simulink model "ee_import_fem_maxwell"  (R2021b)
settings: Solver=FixedStepAuto  StartTime=0.0  StopTime=tsim  FixedStep=Ts  RelTol=1e-3  AbsTol=1e-3
StopFcn:
  | ee_addSimlogTimeStamp(bdroot)
values from neighbouring files (symbols this model uses):
  angleVec = [0 1 2 3 4 5 6 7 8 9 10 11 ... (31 elements, 1x31)]    [matlab.mat]
  data =     [pmsm_phi2i_21p.mat]
  fdVec = Phid_Vec(index_d)    [di_pmsm_model_generator_invLUT_V2.m]    (also in matlab.mat = [-0.2 -0.175 -0.15 -0.125 -0.1 0 0.1 0.15 0.2 0.25 0.3])
  fqVec = Phiq_Vec(index_q)    [di_pmsm_model_generator_invLUT_V2.m]    (also in matlab.mat = [-0.3 -0.24 -0.18 -0.12 -0.09 0 0.09 0.12 0.18 0.24 0.3])
  Id_LUT = Id_perm(:,index_d,index_q)    [di_pmsm_model_generator_invLUT_V2.m]    (also in matlab.mat = [-299.999952118 -299.999957203 -299.999957203 -299.999957203)
  Id_orig = fliplr(data.i_d)    [di_pmsm_model_generator_invLUT_V2.m]
  Iq_LUT = Iq_perm(:,index_d,index_q)    [di_pmsm_model_generator_invLUT_V2.m]    (also in matlab.mat = [-180.584816304 -190.608960928 -197.843546268 -189.111216324)
  Iq_orig = fliplr(-data.i_q)    [di_pmsm_model_generator_invLUT_V2.m]
  J = 0.02    [di_pmsm_model_MPC_ideal_k2.m]    (also in di_pmsm_model_MPC_k1.m; di_pmsm_model_MPC_k2.m; di_pmsm_model_generator_invLUT_V2.m)
  Ld = 0.0013    [di_pmsm_model_MPC_ideal_k2.m]    (also in di_pmsm_model_MPC_k1.m; di_pmsm_model_MPC_k2.m; di_pmsm_model_generator_invLUT_V2.m)
  Lq = 0.0039    [di_pmsm_model_MPC_ideal_k2.m]    (also in di_pmsm_model_MPC_k1.m; di_pmsm_model_MPC_k2.m; di_pmsm_model_generator_invLUT_V2.m)
  omegae = omegae_ref    [di_pmsm_model_MPC_ideal_k2.m]    (also in di_pmsm_model_MPC_k1.m; di_pmsm_model_MPC_k2.m; di_pmsm_model_generator_invLUT_V2.m = N*RPM*2*pi/60)
  PM = 0.1571    [di_pmsm_model_MPC_ideal_k2.m]    (also in di_pmsm_model_MPC_k1.m; di_pmsm_model_MPC_k2.m; di_pmsm_model_generator_invLUT_V2.m)
  R_s = 0.07    [di_pmsm_model_MPC_ideal_k2.m]    (also in di_pmsm_model_MPC_k1.m; di_pmsm_model_MPC_k2.m; di_pmsm_model_generator_invLUT_V2.m)
  RPM = 1000    [di_pmsm_model_generator_invLUT_V2.m]    (also in sim_3f_fcsmpc_k1.m = 3000)
  torque = fliplr(torque)    [param_fcsmpc.m]    (also in sim_3f_fcsmpc_k1.m = tray_sim_par_real(1:param_sim_Nh))
  Torque_orig = fliplr(torque)    [di_pmsm_model_generator_invLUT_V2.m]
  Torque_perm = permute(Torque_orig,[3,1,2])    [di_pmsm_model_generator_invLUT_V2.m]    (also in matlab.mat = [-417.44568224 -399.66222402 -374.4267079 -354.35960705 -348)
undefined symbols (not defined in the file or in its folder): idVec, iqVec, N
CloseFcn:
  | try,close(h1_ee_import_fem_maxwell),end
  | clear h1_ee_import_fem_maxwell
  | clear simlog_ee_import_fem_maxwell
  | clear N RPM Rload
  | clear angleVec idVec iqVec
  | clear flux0 fluxD fluxQ
  | clear torque
Description:
  | Import IPMSM Flux Linkage Data from ANSYS Maxwell
settings Model: Creator=The MathWorks, Inc.  LastModifiedBy=crist
settings SolverCC: AutoScaleAbsTol=off  AlgebraicLoopSolver=TrustRegion
settings DataIOCC: SaveOutput=off  SignalLogging=off  DSMLogging=off  SaveTime=off  ReturnWorkspaceOutputs=off
settings DebuggingCC: SFMachineParentedDataDiag=warning  ArithmeticOperatorsInVariantConditions=warning
settings SFSimCC: SimUseLocalCustomCode=off  CustomCodeUndefinedFunction=UseInterfaceOnly
settings RTWCC: RTWUseLocalCustomCode=off
settings SimscapeCC: SimscapeLogType=all  SimscapeLogName=simlog_ee_import_fem_maxwell  SimscapeLogLimitData=off  SimscapeLogDataHistory=50000

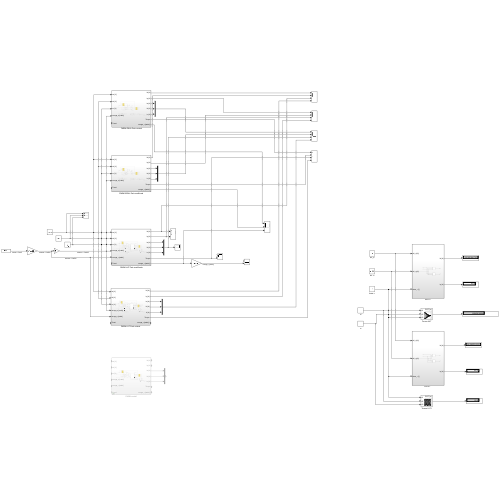
[thumbnail: Simulink's stored preview of the top-level diagram]
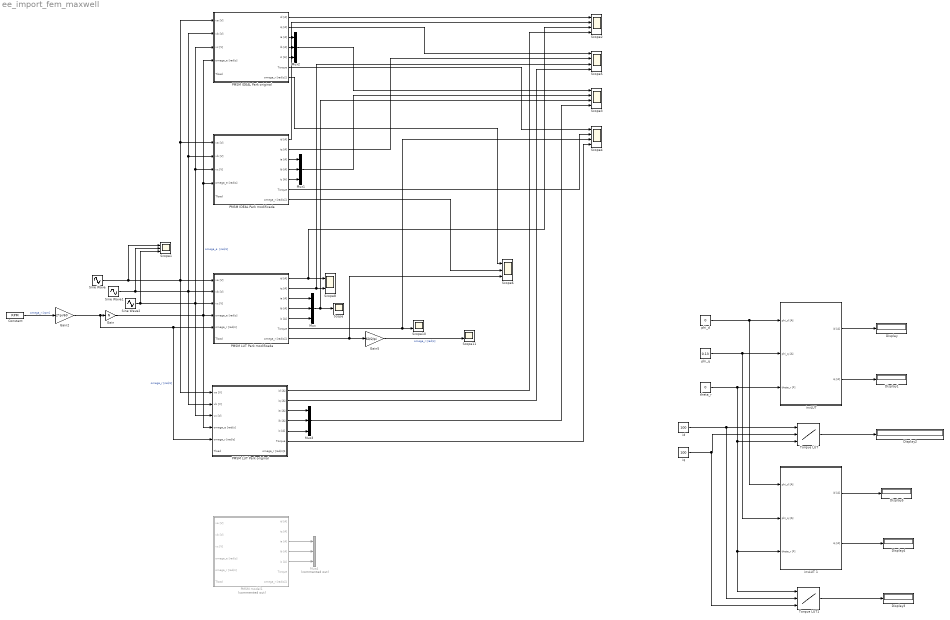
== system ee_import_fem_maxwell ==
  Constant : Constant  Value=RPM
  Display{,1..5} (6 alike) : Display
  Gain : Gain  Gain=N
  Gain2 : Gain  Gain=2*pi/60
  Gain5 : Gain  Gain=60/2/pi
  Mux{,1..3} (4 alike) : Mux  Inputs=3
  Mux4 : Mux  Commented=on  Inputs=3
  PMSM IDEAL Park modificada : Subsystem
  PMSM IDEAL Park original : Subsystem
  PMSM LUT Park modificada : Subsystem
  PMSM LUT Park original : Subsystem
  PMSM model1 : Subsystem  Commented=on
  Scope : Scope
  Scope1 : Scope  NumInputPorts=3
  Scope10 : Scope  NumInputPorts=2
  Scope11 : Scope  NumInputPorts=2
  Scope{2..5} (4 alike) : Scope  NumInputPorts=4
  Scope6 : Scope  NumInputPorts=3
  Scope8 : Scope  NumInputPorts=2
  Sine Wave : Sin  Amplitude=10  Frequency=omegae  Phase=pi/2  SampleTime=0
  Sine Wave1 : Sin  Amplitude=10  Frequency=omegae  Phase=-2*pi/3+pi/2  SampleTime=0
  Sine Wave2 : Sin  Amplitude=10  Frequency=omegae  Phase=-4*pi/3+pi/2  SampleTime=0
  Torque LUT : Lookup_n-D  NumberOfTableDimensions=3  LookupTableObject=iD  BreakpointsForDimension1=idVec  BreakpointsForDimension2=iqVec  BreakpointsForDimension3=angleVec  Table=Torque_orig  InternalRulePriority=Speed  RndMeth=Simplest  InputSameDT=on
      settings: InputPortMap=u0,u1,u2
  Torque LUT1 : Lookup_n-D  NumberOfTableDimensions=3  LookupTableObject=iD  BreakpointsForDimension1=angleVec  BreakpointsForDimension2=idVec  BreakpointsForDimension3=iqVec  Table=Torque_perm  InternalRulePriority=Speed  RndMeth=Simplest  InputSameDT=on
      settings: InputPortMap=u0,u1,u2
  id : Constant  Value=100
  "invLUT " : Subsystem
  invLUT 1 : Subsystem
  iq : Constant  Value=100
  phi_d : Constant  Value=0
  phi_q : Constant  Value=0.13
  theta_r : Constant  Value=0
  wires:
  Gain/1 -> PMSM LUT Park original/4(omega_e [rad/s]), PMSM IDEAL Park modificada/4(omega_e [rad/s]), PMSM IDEAL Park original/4(omega_e [rad/s]), PMSM LUT Park modificada/4(omega_e [rad/s])  "omega_e  [rad/s]"
  Gain2/1 -> PMSM LUT Park original/5(omega_r [rad/s]), PMSM LUT Park modificada/5(omega_r [rad/s]), Gain/1  "omega_r [rad/s]"
  Constant/1 -> Gain2/1  "omega_r [rpm]"
  Sine Wave/1 -> Scope1/1, PMSM LUT Park original/1(va [V]), PMSM IDEAL Park original/1(va [V]), PMSM IDEAL Park modificada/1(va [V]), PMSM LUT Park modificada/1(va [V])
  PMSM LUT Park modificada/3(ia [A]) -> Mux/1
  PMSM LUT Park modificada/4(ib [A]) -> Mux/2
  PMSM LUT Park modificada/5(ic [A]) -> Mux/3
  PMSM LUT Park modificada/6(Torque) -> Scope4/3, Scope10/2
  PMSM LUT Park modificada/7(omega_r [rad/s]1) -> Scope6/3, Gain5/1
  Gain5/1 -> Scope11/2  "omega_r [rad/s]"
  PMSM LUT Park modificada/1(id [A]) -> Scope2/3, Scope8/1
  PMSM LUT Park modificada/2(iq [A]) -> Scope5/3, Scope8/2
  Mux/1 -> Scope3/3, Scope/1
  PMSM IDEAL Park modificada/3(ia [A]) -> Mux1/1
  PMSM IDEAL Park modificada/4(ib [A]) -> Mux1/2
  PMSM IDEAL Park modificada/5(ic [A]) -> Mux1/3
  Sine Wave2/1 -> Scope1/3, PMSM LUT Park original/3(vc [V]), PMSM IDEAL Park original/3(vc [V]), PMSM IDEAL Park modificada/3(vc [V]), PMSM LUT Park modificada/3(vc [V])
  PMSM IDEAL Park original/1(id [A]) -> Scope2/1
  PMSM IDEAL Park modificada/1(id [A]) -> Scope2/2
  PMSM IDEAL Park original/2(iq [A]) -> Scope5/1
  PMSM IDEAL Park modificada/2(iq [A]) -> Scope5/2
  PMSM IDEAL Park original/3(ia [A]) -> Mux2/1
  PMSM IDEAL Park original/4(ib [A]) -> Mux2/2
  PMSM IDEAL Park original/5(ic [A]) -> Mux2/3
  Mux2/1 -> Scope3/1
  Mux1/1 -> Scope3/2
  PMSM IDEAL Park original/6(Torque) -> Scope4/1
  PMSM IDEAL Park modificada/6(Torque) -> Scope4/2
  PMSM IDEAL Park original/7(omega_r [rad/s]1) -> Scope6/1
  PMSM IDEAL Park modificada/7(omega_r [rad/s]1) -> Scope6/2
  PMSM model1/4(ib [A]) -> Mux4/2
  PMSM model1/5(ic [A]) -> Mux4/3
  PMSM model1/3(ia [A]) -> Mux4/1
  Sine Wave1/1 -> Scope1/2, PMSM LUT Park original/2(vb [V]), PMSM IDEAL Park original/2(vb [V]), PMSM IDEAL Park modificada/2(vb [V]), PMSM LUT Park modificada/2(vb [V])
  PMSM LUT Park original/3(ia [A]) -> Mux3/1
  PMSM LUT Park original/4(ib [A]) -> Mux3/2
  PMSM LUT Park original/5(ic [A]) -> Mux3/3
  PMSM LUT Park original/1(id [A]) -> Scope2/4
  PMSM LUT Park original/2(iq [A]) -> Scope5/4
  Mux3/1 -> Scope3/4
  PMSM LUT Park original/6(Torque) -> Scope4/4
  phi_d/1 -> invLUT 1/1(phi_d [A]), "invLUT "/1(phi_d [A])
  phi_q/1 -> "invLUT "/2(phi_q [A]), invLUT 1/2(phi_q [A])
  theta_r/1 -> Torque LUT1/1, invLUT 1/3(theta_r [º]), Torque LUT/3, "invLUT "/3(theta_r [º])
  "invLUT "/1(id [A]) -> Display/1
  "invLUT "/2(iq [A]) -> Display1/1
  Torque LUT/1 -> Display2/1
  Torque LUT1/1 -> Display3/1
  invLUT 1/2(iq [A]) -> Display4/1
  invLUT 1/1(id [A]) -> Display5/1
  id/1 -> Torque LUT1/2, Torque LUT/1
  iq/1 -> Torque LUT1/3, Torque LUT/2

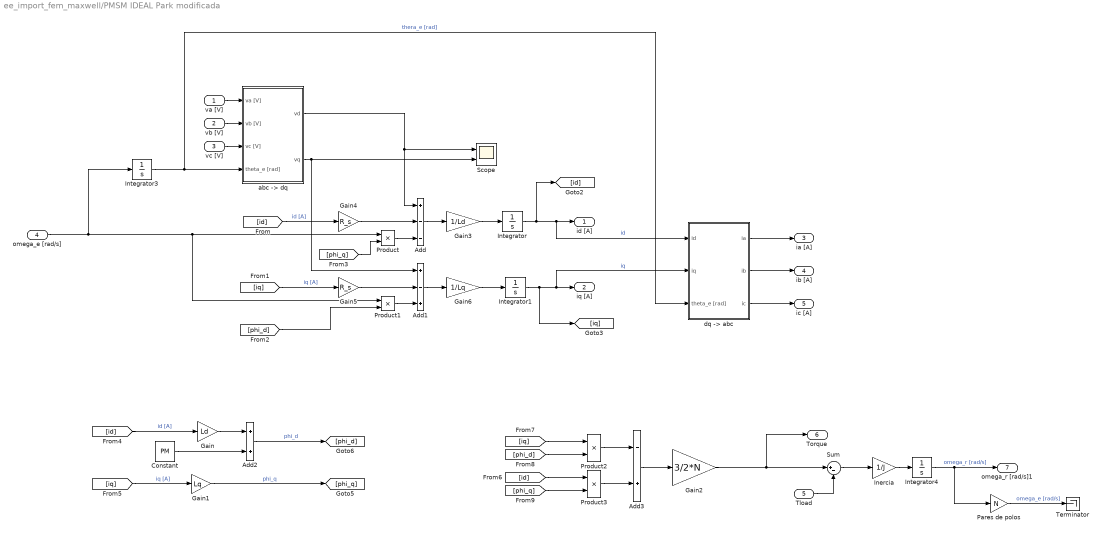
== system ee_import_fem_maxwell/PMSM IDEAL Park modificada ==
  va [V] : Inport
  vb [V] : Inport  Port=2
  vc [V] : Inport  Port=3
  omega_e [rad/s] : Inport  Port=4
  Tload : Inport  Port=5
  Add : Sum  Inputs=+--
  Add1 : Sum  Inputs=+-+
  Add2 : Sum
  Add3 : Sum  Inputs=-+
  Constant : Constant  Value=PM
  Gain : Gain  Gain=Ld
  Gain1 : Gain  Gain=Lq
  Gain2 : Gain  Gain=3/2*N
  Gain3 : Gain  Gain=1/Ld
  Gain4 : Gain  Gain=R_s
  Gain5 : Gain  Gain=R_s
  Gain6 : Gain  Gain=1/Lq
  Inercia : Gain  Gain=1/J
  Integrator : Integrator  InitialCondition=-0.2
  Integrator1 : Integrator
  Integrator3 : Integrator
  Integrator4 : Integrator  InitialCondition=RPM*2*pi/60
  Pares de polos : Gain  Gain=N
  Product{,1..3} (4 alike) : Product
  Scope : Scope  NumInputPorts=2
  Sum : Sum  Inputs=|+-
  Terminator : Terminator
  "abc -> dq" : Subsystem
  "dq -> abc" : Subsystem
  id [A] : Outport
  iq [A] : Outport  Port=2
  ia [A] : Outport  Port=3
  ib [A] : Outport  Port=4
  ic [A] : Outport  Port=5
  Torque : Outport  Port=6
  omega_r [rad/s]1 : Outport  Port=7
  wires:
  Product/1 -> Add/3
  Integrator1/1 -> [iq], "dq -> abc"/2(iq), iq [A]/1  "iq"
  [phi_q] -> Product/2
  omega_e [rad/s]/1 -> Integrator3/1, Product1/1, Product/1
  Add/1 -> Gain3/1
  [id] -> Gain4/1  "id [A]"
  Product1/1 -> Add1/3
  Integrator/1 -> "dq -> abc"/1(id), id [A]/1, [id]  "id"
  Add1/1 -> Gain6/1
  Gain5/1 -> Add1/2
  Gain4/1 -> Add/2
  "abc -> dq"/2(vq) -> Add1/1, Scope/2
  [iq] -> Gain5/1  "iq [A]"
  [phi_d] -> Product1/2
  "abc -> dq"/1(vd) -> Scope/1, Add/1
  va [V]/1 -> "abc -> dq"/1(va [V])
  vb [V]/1 -> "abc -> dq"/2(vb [V])
  vc [V]/1 -> "abc -> dq"/3(vc [V])
  "dq -> abc"/1(ia) -> ia [A]/1
  "dq -> abc"/2(ib) -> ib [A]/1
  "dq -> abc"/3(ic) -> ic [A]/1
  Integrator3/1 -> "abc -> dq"/4(theta_e [rad]), "dq -> abc"/3(theta_e [rad])  "thera_e [rad]"
  Tload/1 -> Sum/2
  Sum/1 -> Inercia/1
  Integrator4/1 -> omega_r [rad/s]1/1, Pares de polos/1  "omega_r [rad/s]"
  Inercia/1 -> Integrator4/1
  Pares de polos/1 -> Terminator/1  "omega_e [rad/s]"
  Gain2/1 -> Sum/1, Torque/1
  Gain/1 -> Add2/1
  Constant/1 -> Add2/2
  [id] -> Gain/1  "id [A]"
  [iq] -> Gain1/1  "iq [A]"
  Add2/1 -> [phi_d]  "phi_d"
  Gain1/1 -> [phi_q]  "phi_q"
  Add3/1 -> Gain2/1
  Product2/1 -> Add3/1
  Product3/1 -> Add3/2
  [id] -> Product3/1
  [iq] -> Product2/1
  [phi_d] -> Product2/2
  [phi_q] -> Product3/2
  Gain3/1 -> Integrator/1
  Gain6/1 -> Integrator1/1

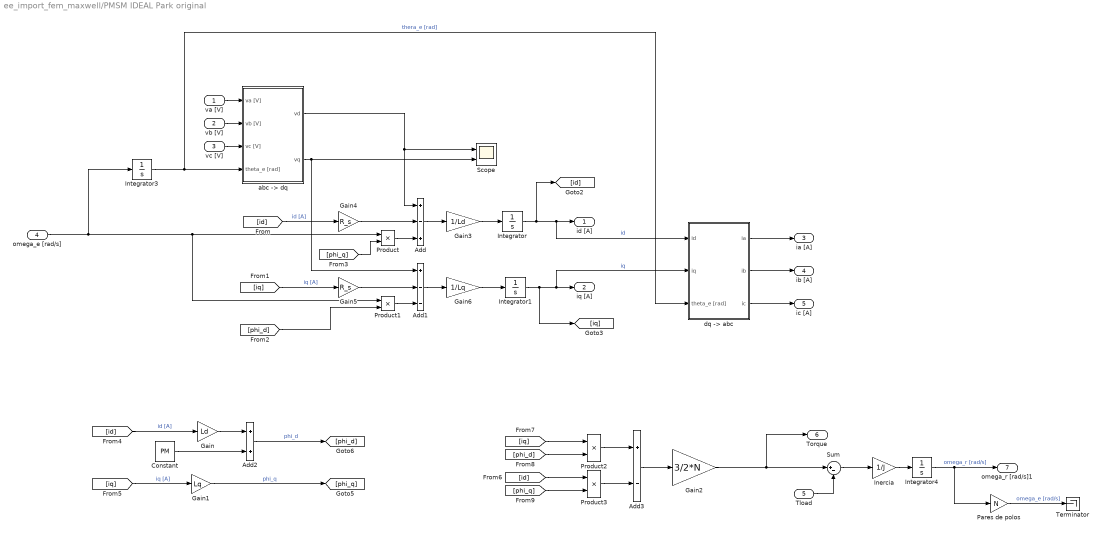
== system ee_import_fem_maxwell/PMSM IDEAL Park original ==
  va [V] : Inport
  vb [V] : Inport  Port=2
  vc [V] : Inport  Port=3
  omega_e [rad/s] : Inport  Port=4
  Tload : Inport  Port=5
  Add : Sum  Inputs=+-+
  Add1 : Sum  Inputs=+--
  Add2 : Sum
  Add3 : Sum  Inputs=+-
  Constant : Constant  Value=PM
  Gain : Gain  Gain=Ld
  Gain1 : Gain  Gain=Lq
  Gain2 : Gain  Gain=3/2*N
  Gain3 : Gain  Gain=1/Ld
  Gain4 : Gain  Gain=R_s
  Gain5 : Gain  Gain=R_s
  Gain6 : Gain  Gain=1/Lq
  Inercia : Gain  Gain=1/J
  Integrator : Integrator  InitialCondition=-0.2
  Integrator1 : Integrator
  Integrator3 : Integrator
  Integrator4 : Integrator  InitialCondition=RPM*2*pi/60
  Pares de polos : Gain  Gain=N
  Product{,1..3} (4 alike) : Product
  Scope : Scope  NumInputPorts=2
  Sum : Sum  Inputs=|+-
  Terminator : Terminator
  "abc -> dq" : Subsystem
  "dq -> abc" : Subsystem
  id [A] : Outport
  iq [A] : Outport  Port=2
  ia [A] : Outport  Port=3
  ib [A] : Outport  Port=4
  ic [A] : Outport  Port=5
  Torque : Outport  Port=6
  omega_r [rad/s]1 : Outport  Port=7
  wires:
  Gain6/1 -> Integrator1/1
  Gain3/1 -> Integrator/1
  [phi_q] -> Product3/2
  [phi_d] -> Product2/2
  [iq] -> Product2/1
  [id] -> Product3/1
  Product3/1 -> Add3/2
  Product2/1 -> Add3/1
  Add3/1 -> Gain2/1
  Gain1/1 -> [phi_q]  "phi_q"
  Add2/1 -> [phi_d]  "phi_d"
  [iq] -> Gain1/1  "iq [A]"
  [id] -> Gain/1  "id [A]"
  Constant/1 -> Add2/2
  Gain/1 -> Add2/1
  Gain2/1 -> Torque/1, Sum/1
  Pares de polos/1 -> Terminator/1  "omega_e [rad/s]"
  Inercia/1 -> Integrator4/1
  Integrator4/1 -> Pares de polos/1, omega_r [rad/s]1/1  "omega_r [rad/s]"
  Sum/1 -> Inercia/1
  Tload/1 -> Sum/2
  Integrator3/1 -> "dq -> abc"/3(theta_e [rad]), "abc -> dq"/4(theta_e [rad])  "thera_e [rad]"
  "dq -> abc"/3(ic) -> ic [A]/1
  "dq -> abc"/2(ib) -> ib [A]/1
  "dq -> abc"/1(ia) -> ia [A]/1
  vc [V]/1 -> "abc -> dq"/3(vc [V])
  vb [V]/1 -> "abc -> dq"/2(vb [V])
  va [V]/1 -> "abc -> dq"/1(va [V])
  "abc -> dq"/1(vd) -> Add/1, Scope/1
  [phi_d] -> Product1/2
  [iq] -> Gain5/1  "iq [A]"
  "abc -> dq"/2(vq) -> Scope/2, Add1/1
  Gain4/1 -> Add/2
  Gain5/1 -> Add1/2
  Add1/1 -> Gain6/1
  Integrator/1 -> [id], id [A]/1, "dq -> abc"/1(id)  "id"
  Product1/1 -> Add1/3
  [id] -> Gain4/1  "id [A]"
  Add/1 -> Gain3/1
  omega_e [rad/s]/1 -> Product/1, Product1/1, Integrator3/1
  [phi_q] -> Product/2
  Integrator1/1 -> iq [A]/1, "dq -> abc"/2(iq), [iq]  "iq"
  Product/1 -> Add/3

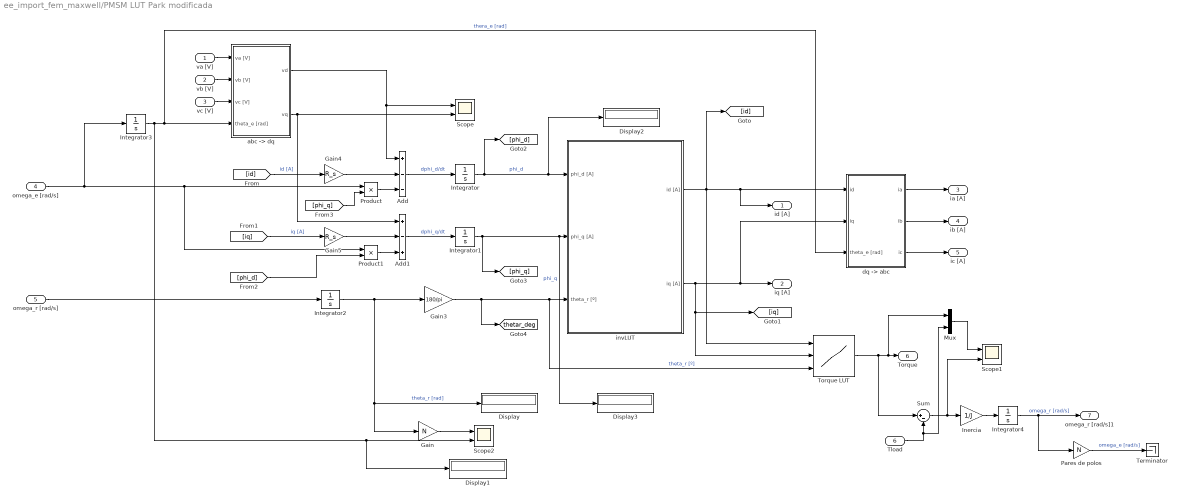
== system ee_import_fem_maxwell/PMSM LUT Park modificada ==
  va [V] : Inport
  vb [V] : Inport  Port=2
  vc [V] : Inport  Port=3
  omega_e [rad/s] : Inport  Port=4
  omega_r [rad/s] : Inport  Port=5
  Tload : Inport  Port=6
  Add : Sum  Inputs=+--
  Add1 : Sum  Inputs=+-+
  Display{,1..3} (4 alike) : Display
  Gain : Gain  Gain=N
  Gain3 : Gain  Gain=180/pi
  Gain4 : Gain  Gain=R_s
  Gain5 : Gain  Gain=R_s
  Inercia : Gain  Gain=1/J
  Integrator : Integrator  InitialCondition=-0.2
  Integrator1 : Integrator
  Integrator2 : Integrator  WrapState=on  WrappedStateUpperValue=2*pi/3/N  WrappedStateLowerValue=0
  Integrator3 : Integrator
  Integrator4 : Integrator  InitialCondition=RPM*2*pi/60
  Mux : Mux  Inputs=2
  Pares de polos : Gain  Gain=N
  Product : Product
  Product1 : Product
  Scope : Scope  NumInputPorts=2
  Scope1 : Scope  NumInputPorts=2
  Scope2 : Scope  NumInputPorts=2
  Sum : Sum  Inputs=|+-
  Terminator : Terminator
  Torque LUT : Lookup_n-D  NumberOfTableDimensions=3  LookupTableObject=iD  BreakpointsForDimension1=idVec  BreakpointsForDimension2=iqVec  BreakpointsForDimension3=angleVec  Table=torque  InternalRulePriority=Speed  RndMeth=Simplest  InputSameDT=on
      settings: InputPortMap=u0,u1,u2
  "abc -> dq" : Subsystem
  "dq -> abc" : Subsystem
  "invLUT " : Subsystem
  id [A] : Outport
  iq [A] : Outport  Port=2
  ia [A] : Outport  Port=3
  ib [A] : Outport  Port=4
  ic [A] : Outport  Port=5
  Torque : Outport  Port=6
  omega_r [rad/s]1 : Outport  Port=7
  tag scope: thetar_deg=global
  wires:
  Product/1 -> Add/3
  Integrator1/1 -> [phi_q], Display3/1, "invLUT "/2(phi_q [A])  "phi_q"
  [phi_q] -> Product/2
  omega_e [rad/s]/1 -> Integrator3/1, Product1/1, Product/1
  Add/1 -> Integrator/1  "dphi_d/dt"
  [id] -> Gain4/1  "id [A]"
  Product1/1 -> Add1/3
  "invLUT "/1(id [A]) -> "dq -> abc"/1(id), id [A]/1, Torque LUT/1, [id]
  Integrator/1 -> Display2/1, "invLUT "/1(phi_d [A]), [phi_d]  "phi_d"
  "invLUT "/2(iq [A]) -> Torque LUT/2, [iq], "dq -> abc"/2(iq), iq [A]/1
  Add1/1 -> Integrator1/1  "dphi_q/dt"
  Gain5/1 -> Add1/2
  Gain4/1 -> Add/2
  "abc -> dq"/2(vq) -> Add1/1, Scope/2
  [iq] -> Gain5/1  "iq [A]"
  [phi_d] -> Product1/2
  "abc -> dq"/1(vd) -> Scope/1, Add/1
  va [V]/1 -> "abc -> dq"/1(va [V])
  vb [V]/1 -> "abc -> dq"/2(vb [V])
  vc [V]/1 -> "abc -> dq"/3(vc [V])
  Gain3/1 -> [thetar_deg], Torque LUT/3, "invLUT "/3(theta_r [º])  "theta_r [º]"
  omega_r [rad/s]/1 -> Integrator2/1
  "dq -> abc"/1(ia) -> ia [A]/1
  "dq -> abc"/2(ib) -> ib [A]/1
  "dq -> abc"/3(ic) -> ic [A]/1
  Integrator2/1 -> Display/1, Gain/1, Gain3/1  "theta_r [rad]"
  Integrator3/1 -> Display1/1, Scope2/2, "dq -> abc"/3(theta_e [rad]), "abc -> dq"/4(theta_e [rad])  "thera_e [rad]"
  Tload/1 -> Mux/2, Sum/2
  Sum/1 -> Scope1/2, Inercia/1
  Integrator4/1 -> omega_r [rad/s]1/1, Pares de polos/1  "omega_r [rad/s]"
  Inercia/1 -> Integrator4/1
  Pares de polos/1 -> Terminator/1  "omega_e [rad/s]"
  Torque LUT/1 -> Sum/1, Mux/1, Torque/1
  Mux/1 -> Scope1/1
  Gain/1 -> Scope2/1

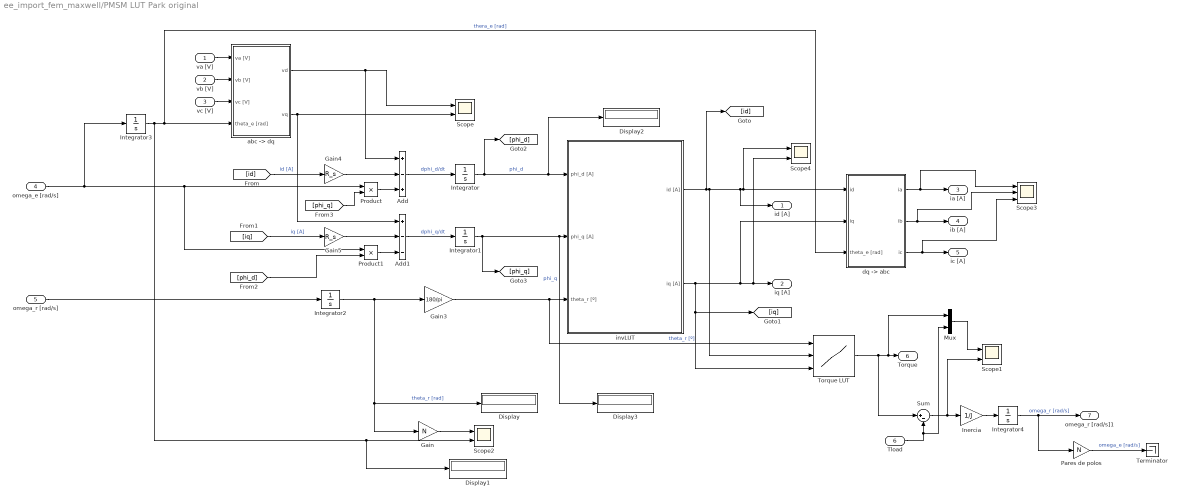
== system ee_import_fem_maxwell/PMSM LUT Park original ==
  va [V] : Inport
  vb [V] : Inport  Port=2
  vc [V] : Inport  Port=3
  omega_e [rad/s] : Inport  Port=4
  omega_r [rad/s] : Inport  Port=5
  Tload : Inport  Port=6
  Add : Sum  Inputs=+-+
  Add1 : Sum  Inputs=+--
  Display{,1..3} (4 alike) : Display
  Gain : Gain  Gain=N
  Gain3 : Gain  Gain=180/pi
  Gain4 : Gain  Gain=R_s
  Gain5 : Gain  Gain=R_s
  Inercia : Gain  Gain=1/J
  Integrator : Integrator  InitialCondition=-0.2
  Integrator1 : Integrator
  Integrator2 : Integrator  WrapState=on  WrappedStateUpperValue=2*pi/3/N  WrappedStateLowerValue=0
  Integrator3 : Integrator
  Integrator4 : Integrator  InitialCondition=RPM*2*pi/60
  Mux : Mux  Inputs=2
  Pares de polos : Gain  Gain=N
  Product : Product
  Product1 : Product
  Scope{,1..2,4} (4 alike) : Scope  NumInputPorts=2
  Scope3 : Scope  NumInputPorts=3
  Sum : Sum  Inputs=|+-
  Terminator : Terminator
  Torque LUT : Lookup_n-D  NumberOfTableDimensions=3  LookupTableObject=iD  BreakpointsForDimension1=angleVec  BreakpointsForDimension2=idVec  BreakpointsForDimension3=iqVec  Table=Torque_perm  InternalRulePriority=Speed  RndMeth=Simplest  InputSameDT=on
      settings: InputPortMap=u0,u1,u2
  "abc -> dq" : Subsystem
  "dq -> abc" : Subsystem
  "invLUT " : Subsystem
  id [A] : Outport
  iq [A] : Outport  Port=2
  ia [A] : Outport  Port=3
  ib [A] : Outport  Port=4
  ic [A] : Outport  Port=5
  Torque : Outport  Port=6
  omega_r [rad/s]1 : Outport  Port=7
  wires:
  Gain/1 -> Scope2/1
  Mux/1 -> Scope1/1
  Torque LUT/1 -> Torque/1, Mux/1, Sum/1
  Pares de polos/1 -> Terminator/1  "omega_e [rad/s]"
  Inercia/1 -> Integrator4/1
  Integrator4/1 -> Pares de polos/1, omega_r [rad/s]1/1  "omega_r [rad/s]"
  Sum/1 -> Inercia/1, Scope1/2
  Tload/1 -> Sum/2, Mux/2
  Integrator3/1 -> "abc -> dq"/4(theta_e [rad]), "dq -> abc"/3(theta_e [rad]), Scope2/2, Display1/1  "thera_e [rad]"
  Integrator2/1 -> Gain3/1, Gain/1, Display/1  "theta_r [rad]"
  "dq -> abc"/3(ic) -> Scope3/3, ic [A]/1
  "dq -> abc"/2(ib) -> Scope3/2, ib [A]/1
  "dq -> abc"/1(ia) -> Scope3/1, ia [A]/1
  omega_r [rad/s]/1 -> Integrator2/1
  Gain3/1 -> Torque LUT/1, "invLUT "/3(theta_r [º])  "theta_r [º]"
  vc [V]/1 -> "abc -> dq"/3(vc [V])
  vb [V]/1 -> "abc -> dq"/2(vb [V])
  va [V]/1 -> "abc -> dq"/1(va [V])
  "abc -> dq"/1(vd) -> Add/1, Scope/1
  [phi_d] -> Product1/2
  [iq] -> Gain5/1  "iq [A]"
  "abc -> dq"/2(vq) -> Scope/2, Add1/1
  Gain4/1 -> Add/2
  Gain5/1 -> Add1/2
  Add1/1 -> Integrator1/1  "dphi_q/dt"
  "invLUT "/2(iq [A]) -> Scope4/2, iq [A]/1, "dq -> abc"/2(iq), Torque LUT/3, [iq]
  Integrator/1 -> [phi_d], "invLUT "/1(phi_d [A]), Display2/1  "phi_d"
  "invLUT "/1(id [A]) -> Scope4/1, "dq -> abc"/1(id), id [A]/1, Torque LUT/2, [id]
  Product1/1 -> Add1/3
  [id] -> Gain4/1  "id [A]"
  Add/1 -> Integrator/1  "dphi_d/dt"
  omega_e [rad/s]/1 -> Product/1, Product1/1, Integrator3/1
  [phi_q] -> Product/2
  Integrator1/1 -> "invLUT "/2(phi_q [A]), Display3/1, [phi_q]  "phi_q"
  Product/1 -> Add/3

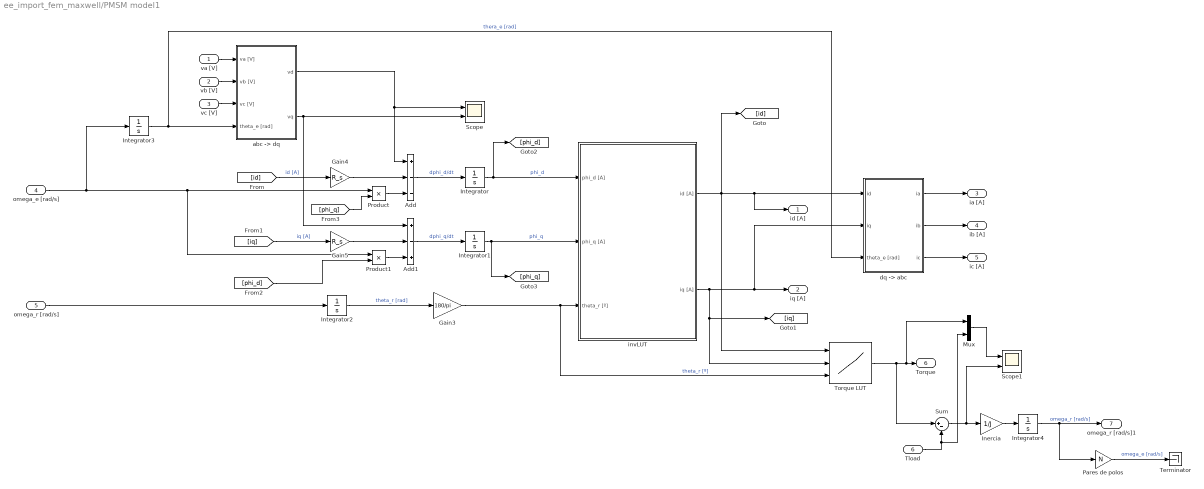
== system ee_import_fem_maxwell/PMSM model1 ==
  va [V] : Inport
  vb [V] : Inport  Port=2
  vc [V] : Inport  Port=3
  omega_e [rad/s] : Inport  Port=4
  omega_r [rad/s] : Inport  Port=5
  Tload : Inport  Port=6
  Add : Sum  Inputs=+--
  Add1 : Sum  Inputs=+-+
  Gain3 : Gain  Gain=180/pi
  Gain4 : Gain  Gain=R_s
  Gain5 : Gain  Gain=R_s
  Inercia : Gain  Gain=1/J
  Integrator : Integrator  InitialCondition=0.1
  Integrator1 : Integrator
  Integrator2 : Integrator  WrapState=on  WrappedStateUpperValue=2*pi/3/N  WrappedStateLowerValue=0
  Integrator3 : Integrator
  Integrator4 : Integrator  InitialCondition=RPM*2*pi/60
  Mux : Mux  Inputs=2
  Pares de polos : Gain  Gain=N
  Product : Product
  Product1 : Product
  Scope : Scope  NumInputPorts=2
  Scope1 : Scope  NumInputPorts=2
  Sum : Sum  Inputs=|+-
  Terminator : Terminator
  Torque LUT : Lookup_n-D  NumberOfTableDimensions=3  LookupTableObject=iD  BreakpointsForDimension1=idVec  BreakpointsForDimension2=iqVec  BreakpointsForDimension3=angleVec  Table=torque  InternalRulePriority=Speed  RndMeth=Simplest  InputSameDT=on
      settings: InputPortMap=u0,u1,u2
  "abc -> dq" : Subsystem
  "dq -> abc" : Subsystem
  "invLUT " : Subsystem
  id [A] : Outport
  iq [A] : Outport  Port=2
  ia [A] : Outport  Port=3
  ib [A] : Outport  Port=4
  ic [A] : Outport  Port=5
  Torque : Outport  Port=6
  omega_r [rad/s]1 : Outport  Port=7
  wires:
  Mux/1 -> Scope1/1
  Torque LUT/1 -> Torque/1, Mux/1, Sum/1
  Pares de polos/1 -> Terminator/1  "omega_e [rad/s]"
  Inercia/1 -> Integrator4/1
  Integrator4/1 -> Pares de polos/1, omega_r [rad/s]1/1  "omega_r [rad/s]"
  Sum/1 -> Inercia/1, Scope1/2
  Tload/1 -> Sum/2, Mux/2
  Integrator3/1 -> "abc -> dq"/4(theta_e [rad]), "dq -> abc"/3(theta_e [rad])  "thera_e [rad]"
  Integrator2/1 -> Gain3/1  "theta_r [rad]"
  "dq -> abc"/3(ic) -> ic [A]/1
  "dq -> abc"/2(ib) -> ib [A]/1
  "dq -> abc"/1(ia) -> ia [A]/1
  omega_r [rad/s]/1 -> Integrator2/1
  Gain3/1 -> "invLUT "/3(theta_r [º]), Torque LUT/3  "theta_r [º]"
  vc [V]/1 -> "abc -> dq"/3(vc [V])
  vb [V]/1 -> "abc -> dq"/2(vb [V])
  va [V]/1 -> "abc -> dq"/1(va [V])
  "abc -> dq"/1(vd) -> Add/1, Scope/1
  [phi_d] -> Product1/2
  [iq] -> Gain5/1  "iq [A]"
  "abc -> dq"/2(vq) -> Scope/2, Add1/1
  Gain4/1 -> Add/2
  Gain5/1 -> Add1/2
  Add1/1 -> Integrator1/1  "dphi_q/dt"
  "invLUT "/2(iq [A]) -> iq [A]/1, "dq -> abc"/2(iq), [iq], Torque LUT/2
  Integrator/1 -> [phi_d], "invLUT "/1(phi_d [A])  "phi_d"
  "invLUT "/1(id [A]) -> [id], Torque LUT/1, id [A]/1, "dq -> abc"/1(id)
  Product1/1 -> Add1/3
  [id] -> Gain4/1  "id [A]"
  Add/1 -> Integrator/1  "dphi_d/dt"
  omega_e [rad/s]/1 -> Product/1, Product1/1, Integrator3/1
  [phi_q] -> Product/2
  Integrator1/1 -> "invLUT "/2(phi_q [A]), [phi_q]  "phi_q"
  Product/1 -> Add/3

== system ee_import_fem_maxwell/invLUT  ==
  phi_d [A] : Inport
  phi_q [A] : Inport  Port=2
  theta_r [º] : Inport  Port=3
  n-D Lookup Table : Lookup_n-D  NumberOfTableDimensions=3  LookupTableObject=iD  BreakpointsForDimension1=data.phi_d  BreakpointsForDimension2=data.phi_q  BreakpointsForDimension3=data.theta  Table=Id_orig  InternalRulePriority=Speed  RndMeth=Simplest  InputSameDT=on
      settings: InputPortMap=u0,u1,u2
  n-D Lookup Table2 : Lookup_n-D  NumberOfTableDimensions=3  LookupTableObject=iD  BreakpointsForDimension1=data.phi_d  BreakpointsForDimension2=data.phi_q  BreakpointsForDimension3=data.theta  Table=Iq_orig  InternalRulePriority=Speed  RndMeth=Simplest  InputSameDT=on
      settings: InputPortMap=u0,u1,u2
  id [A] : Outport
  iq [A] : Outport  Port=2
  wires:
  n-D Lookup Table/1 -> id [A]/1  "id [A]"
  phi_d [A]/1 -> n-D Lookup Table2/1, n-D Lookup Table/1
  phi_q [A]/1 -> n-D Lookup Table2/2, n-D Lookup Table/2
  n-D Lookup Table2/1 -> iq [A]/1  "iq [A]"
  theta_r [º]/1 -> n-D Lookup Table2/3, n-D Lookup Table/3

== system ee_import_fem_maxwell/invLUT 1 ==
  phi_d [A] : Inport
  phi_q [A] : Inport  Port=2
  theta_r [º] : Inport  Port=3
  n-D Lookup Table : Lookup_n-D  NumberOfTableDimensions=3  LookupTableObject=iD  BreakpointsForDimension1=angleVec  BreakpointsForDimension2=fdVec  BreakpointsForDimension3=fqVec  Table=Id_LUT  InternalRulePriority=Speed  RndMeth=Simplest  InputSameDT=on
      settings: InputPortMap=u0,u1,u2
  n-D Lookup Table2 : Lookup_n-D  NumberOfTableDimensions=3  LookupTableObject=iD  BreakpointsForDimension1=angleVec  BreakpointsForDimension2=fdVec  BreakpointsForDimension3=fqVec  Table=Iq_LUT  InternalRulePriority=Speed  RndMeth=Simplest  InputSameDT=on
      settings: InputPortMap=u0,u1,u2
  id [A] : Outport
  iq [A] : Outport  Port=2
  wires:
  theta_r [º]/1 -> n-D Lookup Table2/1, n-D Lookup Table/1
  n-D Lookup Table2/1 -> iq [A]/1  "iq [A]"
  phi_q [A]/1 -> n-D Lookup Table2/3, n-D Lookup Table/3
  phi_d [A]/1 -> n-D Lookup Table2/2, n-D Lookup Table/2
  n-D Lookup Table/1 -> id [A]/1  "id [A]"

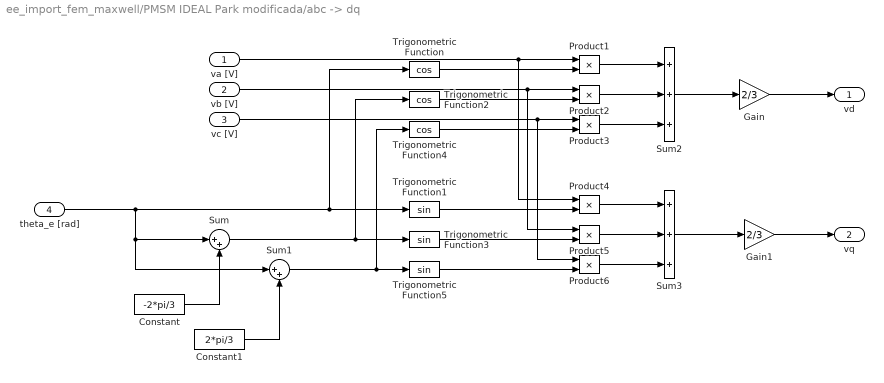
== system ee_import_fem_maxwell/PMSM IDEAL Park modificada/abc -> dq ==
  va [V] : Inport
  vb [V] : Inport  Port=2
  vc [V] : Inport  Port=3
  theta_e [rad] : Inport  Port=4
  Constant : Constant  Value=-2*pi/3
  Constant1 : Constant  Value=2*pi/3
  Gain : Gain  Gain=2/3
  Gain1 : Gain  Gain=2/3
  Product{1..6} (6 alike) : Product  RndMeth=Zero
  Sum : Sum  Inputs=|++
  Sum1 : Sum  Inputs=|++
  Sum2 : Sum  Inputs=+++
  Sum3 : Sum  Inputs=+++
  Trigonometric Function : Trigonometry  Operator=cos
  Trigonometric Function1 : Trigonometry
  Trigonometric Function2 : Trigonometry  Operator=cos
  Trigonometric Function3 : Trigonometry
  Trigonometric Function4 : Trigonometry  Operator=cos
  Trigonometric Function5 : Trigonometry
  vd : Outport
  vq : Outport  Port=2
  wires:
  Gain1/1 -> vq/1
  Gain/1 -> vd/1
  Product1/1 -> Sum2/1
  Trigonometric Function1/1 -> Product4/2
  vb [V]/1 -> Product5/1, Product2/1
  Trigonometric Function/1 -> Product1/2
  theta_e [rad]/1 -> Sum1/1, Sum/1, Trigonometric Function/1, Trigonometric Function1/1
  Sum2/1 -> Gain/1
  Sum3/1 -> Gain1/1
  Constant/1 -> Sum/2
  Constant1/1 -> Sum1/2
  Sum/1 -> Trigonometric Function3/1, Trigonometric Function2/1
  Sum1/1 -> Trigonometric Function4/1, Trigonometric Function5/1
  va [V]/1 -> Product4/1, Product1/1
  Product2/1 -> Sum2/2
  Product3/1 -> Sum2/3
  Product5/1 -> Sum3/2
  Product6/1 -> Sum3/3
  Product4/1 -> Sum3/1
  vc [V]/1 -> Product6/1, Product3/1
  Trigonometric Function2/1 -> Product2/2
  Trigonometric Function4/1 -> Product3/2
  Trigonometric Function3/1 -> Product5/2
  Trigonometric Function5/1 -> Product6/2

== system ee_import_fem_maxwell/PMSM IDEAL Park modificada/dq -> abc ==
  id : Inport
  iq : Inport  Port=2
  theta_e [rad] : Inport  Port=3
  Constant : Constant  Value=-2*pi/3
  Constant1 : Constant  Value=2*pi/3
  Product{1..6} (6 alike) : Product  RndMeth=Zero
  Sum : Sum  Inputs=|++
  Sum1 : Sum  Inputs=|++
  Sum2 : Sum
  Sum3 : Sum
  Sum4 : Sum
  Trigonometric Function : Trigonometry  Operator=cos
  Trigonometric Function1 : Trigonometry
  Trigonometric Function2 : Trigonometry  Operator=cos
  Trigonometric Function3 : Trigonometry
  Trigonometric Function4 : Trigonometry  Operator=cos
  Trigonometric Function5 : Trigonometry
  ia : Outport
  ib : Outport  Port=2
  ic : Outport  Port=3
  wires:
  Trigonometric Function3/1 -> Product5/2
  Trigonometric Function2/1 -> Product4/2
  Product4/1 -> Sum3/1
  Product5/1 -> Sum3/2
  Product2/1 -> Sum2/2
  id/1 -> Product1/1, Product3/1, Product4/1
  Sum1/1 -> Trigonometric Function5/1, Trigonometric Function4/1
  Sum/1 -> Trigonometric Function3/1, Trigonometric Function2/1
  Constant1/1 -> Sum1/2
  Constant/1 -> Sum/2
  theta_e [rad]/1 -> Sum/1, Sum1/1, Trigonometric Function1/1, Trigonometric Function/1
  Trigonometric Function/1 -> Product1/2
  iq/1 -> Product2/1, Product6/1, Product5/1
  Trigonometric Function1/1 -> Product2/2
  Product1/1 -> Sum2/1
  Sum2/1 -> ia/1
  Sum3/1 -> ib/1
  Sum4/1 -> ic/1
  Product6/1 -> Sum4/2
  Product3/1 -> Sum4/1
  Trigonometric Function4/1 -> Product3/2
  Trigonometric Function5/1 -> Product6/2

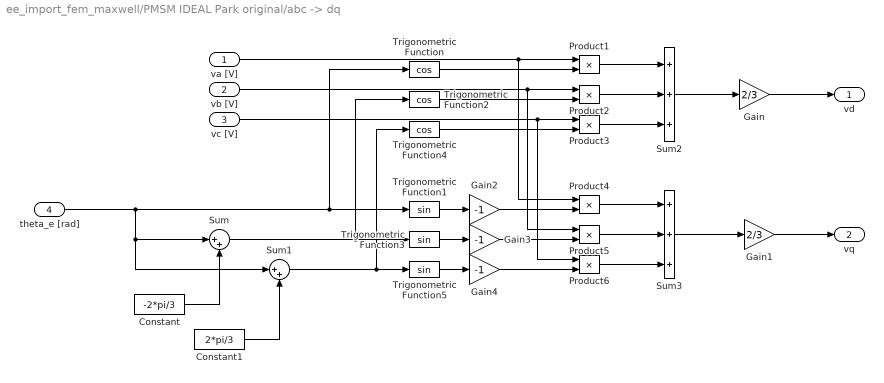
== system ee_import_fem_maxwell/PMSM IDEAL Park original/abc -> dq ==
  va [V] : Inport
  vb [V] : Inport  Port=2
  vc [V] : Inport  Port=3
  theta_e [rad] : Inport  Port=4
  Constant : Constant  Value=-2*pi/3
  Constant1 : Constant  Value=2*pi/3
  Gain : Gain  Gain=2/3
  Gain1 : Gain  Gain=2/3
  Gain2 : Gain  Gain=-1
  Gain3 : Gain  Gain=-1
  Gain4 : Gain  Gain=-1
  Product{1..6} (6 alike) : Product  RndMeth=Zero
  Sum : Sum  Inputs=|++
  Sum1 : Sum  Inputs=|++
  Sum2 : Sum  Inputs=+++
  Sum3 : Sum  Inputs=+++
  Trigonometric Function : Trigonometry  Operator=cos
  Trigonometric Function1 : Trigonometry
  Trigonometric Function2 : Trigonometry  Operator=cos
  Trigonometric Function3 : Trigonometry
  Trigonometric Function4 : Trigonometry  Operator=cos
  Trigonometric Function5 : Trigonometry
  vd : Outport
  vq : Outport  Port=2
  wires:
  Trigonometric Function5/1 -> Gain4/1
  Trigonometric Function3/1 -> Gain3/1
  Trigonometric Function4/1 -> Product3/2
  Trigonometric Function2/1 -> Product2/2
  vc [V]/1 -> Product3/1, Product6/1
  Product4/1 -> Sum3/1
  Product6/1 -> Sum3/3
  Product5/1 -> Sum3/2
  Product3/1 -> Sum2/3
  Product2/1 -> Sum2/2
  va [V]/1 -> Product1/1, Product4/1
  Sum1/1 -> Trigonometric Function5/1, Trigonometric Function4/1
  Sum/1 -> Trigonometric Function2/1, Trigonometric Function3/1
  Constant1/1 -> Sum1/2
  Constant/1 -> Sum/2
  Sum3/1 -> Gain1/1
  Sum2/1 -> Gain/1
  theta_e [rad]/1 -> Trigonometric Function1/1, Trigonometric Function/1, Sum/1, Sum1/1
  Trigonometric Function/1 -> Product1/2
  vb [V]/1 -> Product2/1, Product5/1
  Trigonometric Function1/1 -> Gain2/1
  Product1/1 -> Sum2/1
  Gain/1 -> vd/1
  Gain1/1 -> vq/1
  Gain2/1 -> Product4/2
  Gain3/1 -> Product5/2
  Gain4/1 -> Product6/2

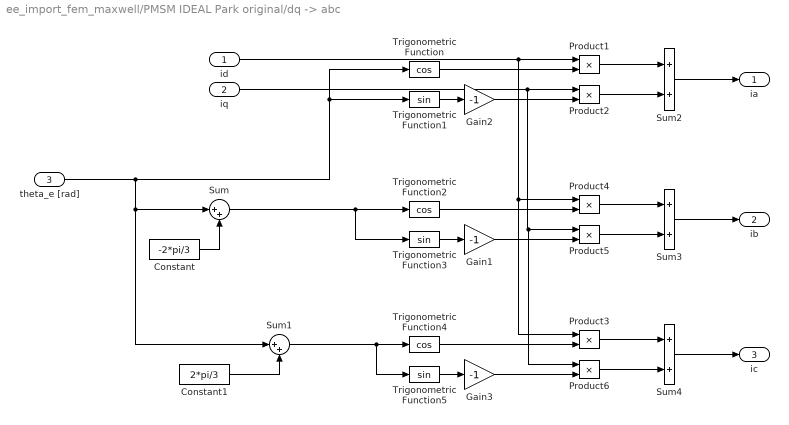
== system ee_import_fem_maxwell/PMSM IDEAL Park original/dq -> abc ==
  id : Inport
  iq : Inport  Port=2
  theta_e [rad] : Inport  Port=3
  Constant : Constant  Value=-2*pi/3
  Constant1 : Constant  Value=2*pi/3
  Gain1 : Gain  Gain=-1
  Gain2 : Gain  Gain=-1
  Gain3 : Gain  Gain=-1
  Product{1..6} (6 alike) : Product  RndMeth=Zero
  Sum : Sum  Inputs=|++
  Sum1 : Sum  Inputs=|++
  Sum2 : Sum
  Sum3 : Sum
  Sum4 : Sum
  Trigonometric Function : Trigonometry  Operator=cos
  Trigonometric Function1 : Trigonometry
  Trigonometric Function2 : Trigonometry  Operator=cos
  Trigonometric Function3 : Trigonometry
  Trigonometric Function4 : Trigonometry  Operator=cos
  Trigonometric Function5 : Trigonometry
  ia : Outport
  ib : Outport  Port=2
  ic : Outport  Port=3
  wires:
  Trigonometric Function5/1 -> Gain3/1
  Trigonometric Function4/1 -> Product3/2
  Product3/1 -> Sum4/1
  Product6/1 -> Sum4/2
  Sum4/1 -> ic/1
  Sum3/1 -> ib/1
  Sum2/1 -> ia/1
  Product1/1 -> Sum2/1
  Trigonometric Function1/1 -> Gain2/1
  iq/1 -> Product5/1, Product6/1, Product2/1
  Trigonometric Function/1 -> Product1/2
  theta_e [rad]/1 -> Trigonometric Function/1, Trigonometric Function1/1, Sum1/1, Sum/1
  Constant/1 -> Sum/2
  Constant1/1 -> Sum1/2
  Sum/1 -> Trigonometric Function2/1, Trigonometric Function3/1
  Sum1/1 -> Trigonometric Function4/1, Trigonometric Function5/1
  id/1 -> Product4/1, Product3/1, Product1/1
  Product2/1 -> Sum2/2
  Product5/1 -> Sum3/2
  Product4/1 -> Sum3/1
  Trigonometric Function2/1 -> Product4/2
  Trigonometric Function3/1 -> Gain1/1
  Gain2/1 -> Product2/2
  Gain1/1 -> Product5/2
  Gain3/1 -> Product6/2

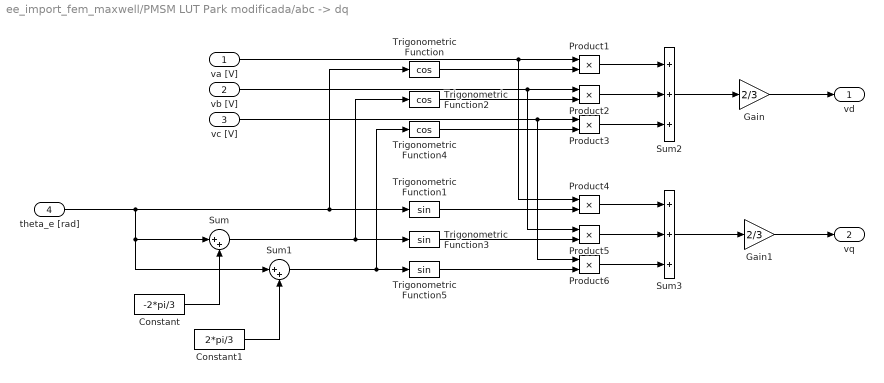
== system ee_import_fem_maxwell/PMSM LUT Park modificada/abc -> dq ==
  va [V] : Inport
  vb [V] : Inport  Port=2
  vc [V] : Inport  Port=3
  theta_e [rad] : Inport  Port=4
  Constant : Constant  Value=-2*pi/3
  Constant1 : Constant  Value=2*pi/3
  Gain : Gain  Gain=2/3
  Gain1 : Gain  Gain=2/3
  Product{1..6} (6 alike) : Product  RndMeth=Zero
  Sum : Sum  Inputs=|++
  Sum1 : Sum  Inputs=|++
  Sum2 : Sum  Inputs=+++
  Sum3 : Sum  Inputs=+++
  Trigonometric Function : Trigonometry  Operator=cos
  Trigonometric Function1 : Trigonometry
  Trigonometric Function2 : Trigonometry  Operator=cos
  Trigonometric Function3 : Trigonometry
  Trigonometric Function4 : Trigonometry  Operator=cos
  Trigonometric Function5 : Trigonometry
  vd : Outport
  vq : Outport  Port=2
  wires:
  Gain1/1 -> vq/1
  Gain/1 -> vd/1
  Product1/1 -> Sum2/1
  Trigonometric Function1/1 -> Product4/2
  vb [V]/1 -> Product5/1, Product2/1
  Trigonometric Function/1 -> Product1/2
  theta_e [rad]/1 -> Sum1/1, Sum/1, Trigonometric Function/1, Trigonometric Function1/1
  Sum2/1 -> Gain/1
  Sum3/1 -> Gain1/1
  Constant/1 -> Sum/2
  Constant1/1 -> Sum1/2
  Sum/1 -> Trigonometric Function3/1, Trigonometric Function2/1
  Sum1/1 -> Trigonometric Function4/1, Trigonometric Function5/1
  va [V]/1 -> Product4/1, Product1/1
  Product2/1 -> Sum2/2
  Product3/1 -> Sum2/3
  Product5/1 -> Sum3/2
  Product6/1 -> Sum3/3
  Product4/1 -> Sum3/1
  vc [V]/1 -> Product6/1, Product3/1
  Trigonometric Function2/1 -> Product2/2
  Trigonometric Function4/1 -> Product3/2
  Trigonometric Function3/1 -> Product5/2
  Trigonometric Function5/1 -> Product6/2

== system ee_import_fem_maxwell/PMSM LUT Park modificada/dq -> abc ==
  id : Inport
  iq : Inport  Port=2
  theta_e [rad] : Inport  Port=3
  Constant : Constant  Value=-2*pi/3
  Constant1 : Constant  Value=2*pi/3
  Product{1..6} (6 alike) : Product  RndMeth=Zero
  Sum : Sum  Inputs=|++
  Sum1 : Sum  Inputs=|++
  Sum2 : Sum
  Sum3 : Sum
  Sum4 : Sum
  Trigonometric Function : Trigonometry  Operator=cos
  Trigonometric Function1 : Trigonometry
  Trigonometric Function2 : Trigonometry  Operator=cos
  Trigonometric Function3 : Trigonometry
  Trigonometric Function4 : Trigonometry  Operator=cos
  Trigonometric Function5 : Trigonometry
  ia : Outport
  ib : Outport  Port=2
  ic : Outport  Port=3
  wires:
  Trigonometric Function3/1 -> Product5/2
  Trigonometric Function2/1 -> Product4/2
  Product4/1 -> Sum3/1
  Product5/1 -> Sum3/2
  Product2/1 -> Sum2/2
  id/1 -> Product1/1, Product3/1, Product4/1
  Sum1/1 -> Trigonometric Function5/1, Trigonometric Function4/1
  Sum/1 -> Trigonometric Function3/1, Trigonometric Function2/1
  Constant1/1 -> Sum1/2
  Constant/1 -> Sum/2
  theta_e [rad]/1 -> Sum/1, Sum1/1, Trigonometric Function1/1, Trigonometric Function/1
  Trigonometric Function/1 -> Product1/2
  iq/1 -> Product2/1, Product6/1, Product5/1
  Trigonometric Function1/1 -> Product2/2
  Product1/1 -> Sum2/1
  Sum2/1 -> ia/1
  Sum3/1 -> ib/1
  Sum4/1 -> ic/1
  Product6/1 -> Sum4/2
  Product3/1 -> Sum4/1
  Trigonometric Function4/1 -> Product3/2
  Trigonometric Function5/1 -> Product6/2

== system ee_import_fem_maxwell/PMSM LUT Park modificada/invLUT  ==
  phi_d [A] : Inport
  phi_q [A] : Inport  Port=2
  theta_r [º] : Inport  Port=3
  n-D Lookup Table : Lookup_n-D  NumberOfTableDimensions=3  LookupTableObject=iD  BreakpointsForDimension1=data.phi_d  BreakpointsForDimension2=data.phi_q  BreakpointsForDimension3=data.theta  Table=data.i_d  InternalRulePriority=Speed  RndMeth=Simplest  InputSameDT=on
      settings: InputPortMap=u0,u1,u2
  n-D Lookup Table2 : Lookup_n-D  NumberOfTableDimensions=3  LookupTableObject=iD  BreakpointsForDimension1=data.phi_d  BreakpointsForDimension2=data.phi_q  BreakpointsForDimension3=data.theta  Table=data.i_q  InternalRulePriority=Speed  RndMeth=Simplest  InputSameDT=on
      settings: InputPortMap=u0,u1,u2
  id [A] : Outport
  iq [A] : Outport  Port=2
  wires:
  n-D Lookup Table/1 -> id [A]/1  "id [A]"
  phi_d [A]/1 -> n-D Lookup Table2/1, n-D Lookup Table/1
  phi_q [A]/1 -> n-D Lookup Table2/2, n-D Lookup Table/2
  n-D Lookup Table2/1 -> iq [A]/1  "iq [A]"
  theta_r [º]/1 -> n-D Lookup Table2/3, n-D Lookup Table/3

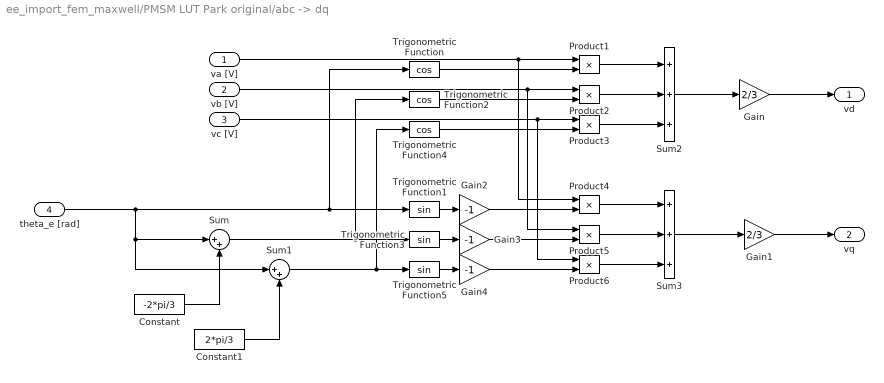
== system ee_import_fem_maxwell/PMSM LUT Park original/abc -> dq ==
  va [V] : Inport
  vb [V] : Inport  Port=2
  vc [V] : Inport  Port=3
  theta_e [rad] : Inport  Port=4
  Constant : Constant  Value=-2*pi/3
  Constant1 : Constant  Value=2*pi/3
  Gain : Gain  Gain=2/3
  Gain1 : Gain  Gain=2/3
  Gain2 : Gain  Gain=-1
  Gain3 : Gain  Gain=-1
  Gain4 : Gain  Gain=-1
  Product{1..6} (6 alike) : Product  RndMeth=Zero
  Sum : Sum  Inputs=|++
  Sum1 : Sum  Inputs=|++
  Sum2 : Sum  Inputs=+++
  Sum3 : Sum  Inputs=+++
  Trigonometric Function : Trigonometry  Operator=cos
  Trigonometric Function1 : Trigonometry
  Trigonometric Function2 : Trigonometry  Operator=cos
  Trigonometric Function3 : Trigonometry
  Trigonometric Function4 : Trigonometry  Operator=cos
  Trigonometric Function5 : Trigonometry
  vd : Outport
  vq : Outport  Port=2
  wires:
  Trigonometric Function5/1 -> Gain4/1
  Trigonometric Function3/1 -> Gain3/1
  Trigonometric Function4/1 -> Product3/2
  Trigonometric Function2/1 -> Product2/2
  vc [V]/1 -> Product3/1, Product6/1
  Product4/1 -> Sum3/1
  Product6/1 -> Sum3/3
  Product5/1 -> Sum3/2
  Product3/1 -> Sum2/3
  Product2/1 -> Sum2/2
  va [V]/1 -> Product1/1, Product4/1
  Sum1/1 -> Trigonometric Function5/1, Trigonometric Function4/1
  Sum/1 -> Trigonometric Function2/1, Trigonometric Function3/1
  Constant1/1 -> Sum1/2
  Constant/1 -> Sum/2
  Sum3/1 -> Gain1/1
  Sum2/1 -> Gain/1
  theta_e [rad]/1 -> Trigonometric Function1/1, Trigonometric Function/1, Sum/1, Sum1/1
  Trigonometric Function/1 -> Product1/2
  vb [V]/1 -> Product2/1, Product5/1
  Trigonometric Function1/1 -> Gain2/1
  Product1/1 -> Sum2/1
  Gain/1 -> vd/1
  Gain1/1 -> vq/1
  Gain2/1 -> Product4/2
  Gain3/1 -> Product5/2
  Gain4/1 -> Product6/2

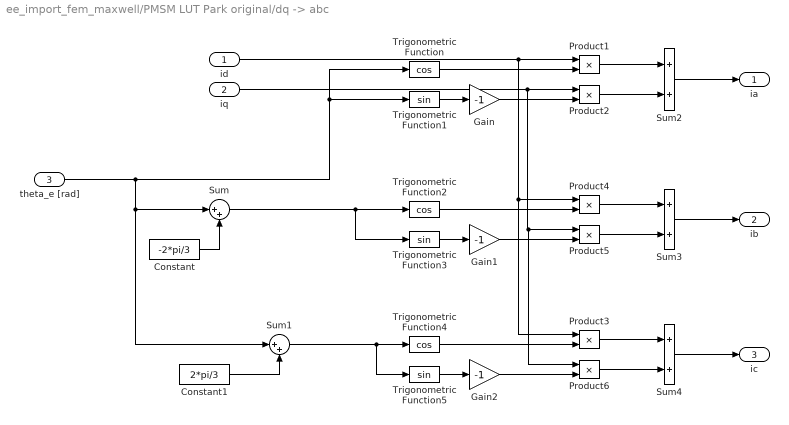
== system ee_import_fem_maxwell/PMSM LUT Park original/dq -> abc ==
  id : Inport
  iq : Inport  Port=2
  theta_e [rad] : Inport  Port=3
  Constant : Constant  Value=-2*pi/3
  Constant1 : Constant  Value=2*pi/3
  Gain : Gain  Gain=-1
  Gain1 : Gain  Gain=-1
  Gain2 : Gain  Gain=-1
  Product{1..6} (6 alike) : Product  RndMeth=Zero
  Sum : Sum  Inputs=|++
  Sum1 : Sum  Inputs=|++
  Sum2 : Sum
  Sum3 : Sum
  Sum4 : Sum
  Trigonometric Function : Trigonometry  Operator=cos
  Trigonometric Function1 : Trigonometry
  Trigonometric Function2 : Trigonometry  Operator=cos
  Trigonometric Function3 : Trigonometry
  Trigonometric Function4 : Trigonometry  Operator=cos
  Trigonometric Function5 : Trigonometry
  ia : Outport
  ib : Outport  Port=2
  ic : Outport  Port=3
  wires:
  Trigonometric Function5/1 -> Gain2/1
  Trigonometric Function4/1 -> Product3/2
  Product3/1 -> Sum4/1
  Product6/1 -> Sum4/2
  Sum4/1 -> ic/1
  Sum3/1 -> ib/1
  Sum2/1 -> ia/1
  Product1/1 -> Sum2/1
  Trigonometric Function1/1 -> Gain/1
  iq/1 -> Product5/1, Product6/1, Product2/1
  Trigonometric Function/1 -> Product1/2
  theta_e [rad]/1 -> Trigonometric Function/1, Trigonometric Function1/1, Sum1/1, Sum/1
  Constant/1 -> Sum/2
  Constant1/1 -> Sum1/2
  Sum/1 -> Trigonometric Function2/1, Trigonometric Function3/1
  Sum1/1 -> Trigonometric Function4/1, Trigonometric Function5/1
  id/1 -> Product4/1, Product3/1, Product1/1
  Product2/1 -> Sum2/2
  Product5/1 -> Sum3/2
  Product4/1 -> Sum3/1
  Trigonometric Function2/1 -> Product4/2
  Trigonometric Function3/1 -> Gain1/1
  Gain/1 -> Product2/2
  Gain1/1 -> Product5/2
  Gain2/1 -> Product6/2

== system ee_import_fem_maxwell/PMSM LUT Park original/invLUT  ==
  phi_d [A] : Inport
  phi_q [A] : Inport  Port=2
  theta_r [º] : Inport  Port=3
  n-D Lookup Table : Lookup_n-D  NumberOfTableDimensions=3  LookupTableObject=iD  BreakpointsForDimension1=angleVec  BreakpointsForDimension2=fdVec  BreakpointsForDimension3=fqVec  Table=Id_LUT  InternalRulePriority=Speed  RndMeth=Simplest  InputSameDT=on
      settings: InputPortMap=u0,u1,u2
  n-D Lookup Table2 : Lookup_n-D  NumberOfTableDimensions=3  LookupTableObject=iD  BreakpointsForDimension1=angleVec  BreakpointsForDimension2=fdVec  BreakpointsForDimension3=fqVec  Table=Iq_LUT  InternalRulePriority=Speed  RndMeth=Simplest  InputSameDT=on
      settings: InputPortMap=u0,u1,u2
  id [A] : Outport
  iq [A] : Outport  Port=2
  wires:
  theta_r [º]/1 -> n-D Lookup Table/1, n-D Lookup Table2/1
  n-D Lookup Table2/1 -> iq [A]/1  "iq [A]"
  phi_q [A]/1 -> n-D Lookup Table2/3, n-D Lookup Table/3
  phi_d [A]/1 -> n-D Lookup Table2/2, n-D Lookup Table/2
  n-D Lookup Table/1 -> id [A]/1  "id [A]"

== system ee_import_fem_maxwell/PMSM model1/abc -> dq ==
  va [V] : Inport
  vb [V] : Inport  Port=2
  vc [V] : Inport  Port=3
  theta_e [rad] : Inport  Port=4
  Constant : Constant  Value=-2*pi/3
  Constant1 : Constant  Value=2*pi/3
  Gain : Gain  Gain=2/3
  Gain1 : Gain  Gain=2/3
  Product{1..6} (6 alike) : Product  RndMeth=Zero
  Sum : Sum  Inputs=|++
  Sum1 : Sum  Inputs=|++
  Sum2 : Sum  Inputs=+++
  Sum3 : Sum  Inputs=+++
  Trigonometric Function : Trigonometry  Operator=cos
  Trigonometric Function1 : Trigonometry
  Trigonometric Function2 : Trigonometry  Operator=cos
  Trigonometric Function3 : Trigonometry
  Trigonometric Function4 : Trigonometry  Operator=cos
  Trigonometric Function5 : Trigonometry
  vd : Outport
  vq : Outport  Port=2
  wires:
  Trigonometric Function5/1 -> Product6/2
  Trigonometric Function3/1 -> Product5/2
  Trigonometric Function4/1 -> Product3/2
  Trigonometric Function2/1 -> Product2/2
  vc [V]/1 -> Product3/1, Product6/1
  Product4/1 -> Sum3/1
  Product6/1 -> Sum3/3
  Product5/1 -> Sum3/2
  Product3/1 -> Sum2/3
  Product2/1 -> Sum2/2
  va [V]/1 -> Product1/1, Product4/1
  Sum1/1 -> Trigonometric Function5/1, Trigonometric Function4/1
  Sum/1 -> Trigonometric Function2/1, Trigonometric Function3/1
  Constant1/1 -> Sum1/2
  Constant/1 -> Sum/2
  Sum3/1 -> Gain1/1
  Sum2/1 -> Gain/1
  theta_e [rad]/1 -> Trigonometric Function1/1, Trigonometric Function/1, Sum/1, Sum1/1
  Trigonometric Function/1 -> Product1/2
  vb [V]/1 -> Product2/1, Product5/1
  Trigonometric Function1/1 -> Product4/2
  Product1/1 -> Sum2/1
  Gain/1 -> vd/1
  Gain1/1 -> vq/1

== system ee_import_fem_maxwell/PMSM model1/dq -> abc ==
  id : Inport
  iq : Inport  Port=2
  theta_e [rad] : Inport  Port=3
  Constant : Constant  Value=-2*pi/3
  Constant1 : Constant  Value=2*pi/3
  Product{1..6} (6 alike) : Product  RndMeth=Zero
  Sum : Sum  Inputs=|++
  Sum1 : Sum  Inputs=|++
  Sum2 : Sum
  Sum3 : Sum
  Sum4 : Sum
  Trigonometric Function : Trigonometry  Operator=cos
  Trigonometric Function1 : Trigonometry
  Trigonometric Function2 : Trigonometry  Operator=cos
  Trigonometric Function3 : Trigonometry
  Trigonometric Function4 : Trigonometry  Operator=cos
  Trigonometric Function5 : Trigonometry
  ia : Outport
  ib : Outport  Port=2
  ic : Outport  Port=3
  wires:
  Trigonometric Function5/1 -> Product6/2
  Trigonometric Function4/1 -> Product3/2
  Product3/1 -> Sum4/1
  Product6/1 -> Sum4/2
  Sum4/1 -> ic/1
  Sum3/1 -> ib/1
  Sum2/1 -> ia/1
  Product1/1 -> Sum2/1
  Trigonometric Function1/1 -> Product2/2
  iq/1 -> Product5/1, Product6/1, Product2/1
  Trigonometric Function/1 -> Product1/2
  theta_e [rad]/1 -> Trigonometric Function/1, Trigonometric Function1/1, Sum1/1, Sum/1
  Constant/1 -> Sum/2
  Constant1/1 -> Sum1/2
  Sum/1 -> Trigonometric Function2/1, Trigonometric Function3/1
  Sum1/1 -> Trigonometric Function4/1, Trigonometric Function5/1
  id/1 -> Product4/1, Product3/1, Product1/1
  Product2/1 -> Sum2/2
  Product5/1 -> Sum3/2
  Product4/1 -> Sum3/1
  Trigonometric Function2/1 -> Product4/2
  Trigonometric Function3/1 -> Product5/2

== system ee_import_fem_maxwell/PMSM model1/invLUT  ==
  phi_d [A] : Inport
  phi_q [A] : Inport  Port=2
  theta_r [º] : Inport  Port=3
  MATLAB Function2 : MATLAB Function  TreatAsAtomicUnit=on
  MATLAB Function3 : MATLAB Function  TreatAsAtomicUnit=on
  id [A] : Outport
  iq [A] : Outport  Port=2
  wires:
  theta_r [º]/1 -> MATLAB Function3/3(z), MATLAB Function2/3(z)
  MATLAB Function3/1(iq_interp) -> iq [A]/1  "iq [A]"
  phi_q [A]/1 -> MATLAB Function3/2(y), MATLAB Function2/2(y)
  phi_d [A]/1 -> MATLAB Function3/1(x), MATLAB Function2/1(x)
  MATLAB Function2/1(id_interp) -> id [A]/1  "id [A]"

== matlab function ee_import_fem_maxwell/PMSM model1/invLUT /MATLAB Function2 ==
  data: x input; id_interp output; y input; z input; data parameter
function id_interp = fcn(x,y,z,data)

iD = data.i_d;
% iQ = data.i_q;
fD = data.phi_d;
fQ = data.phi_d;
TH = data.theta;

% Buscamos los vértices del cubo
if x<fD(1)
    index_x0 = 1;
    index_x1 = 1;
elseif x>fD(end)
    index_x0 = length(fD);
    index_x1 = length(fD);
else
    x_aux = find(fD <= x);
    index_x0 = x_aux(end);
    index_x1 = x_aux(end)+1;
end
x_0 = fD(index_x0);
x_1 = fD(index_x1);

if y<fQ(1)
    index_y0 = 1;
    index_y1 = 1;
elseif y>fQ(end)
    index_y0 = length(fQ);
    index_y1 = length(fQ);
else
    y_aux = find(fQ <= y);
    index_y0 = y_aux(end);
    index_y1 = y_aux(end)+1;
end
y_0 = fQ(index_y0);
y_1 = fQ(index_y1);

if z<TH(1)
    index_z0 = 1;
    index_z1 = 1;
elseif z>TH(end)
    index_z0 = length(TH);
    index_z1 = length(TH);
else
    z_aux = find(TH <= z);
    index_z0 = z_aux(end);
    index_z1 = z_aux(end)+1;
end
z_0 = TH(index_z0);
z_1 = TH(index_z1);

C_000 = iD(index_x0, index_y0, index_z0);
C_001 = iD(index_x0, index_y0, index_z1);
C_010 = iD(index_x0, index_y1, index_z0);
C_011 = iD(index_x0, index_y1, index_z1);
C_100 = iD(index_x1, index_y0, index_z0);
C_101 = iD(index_x1, index_y0, index_z1);
C_110 = iD(index_x1, index_y1, index_z0);
C_111 = iD(index_x1, index_y1, index_z1);

a_0 = (-C_000*x_1*y_1*z_1 + C_001*x_1*y_1*z_0 + C_010*x_1*y_0*z_1 - C_011*x_1*y_0*z_0 + C_100*x_0*y_1*z_1 - C_101*x_0*y_1*z_0 - C_110*x_0*y_0*z_1 + C_111*x_0*y_0*z_0)/(x_0*y_0*z_0 - x_0*y_0*z_1 - x_0*y_1*z_0 + x_0*y_1*z_1 - x_1*y_0*z_0 + x_1*y_0*z_1 + x_1*y_1*z_0 - x_1*y_1*z_1);
a_1 = (C_000*y_1*z_1 - C_001*y_1*z_0 - C_010*y_0*z_1 + C_011*y_0*z_0 - C_100*y_1*z_1 + C_101*y_1*z_0 + C_110*y_0*z_1 - C_111*y_0*z_0)/(x_0*y_0*z_0 - x_0*y_0*z_1 - x_0*y_1*z_0 + x_0*y_1*z_1 - x_1*y_0*z_0 + x_1*y_0*z_1 + x_1*y_1*z_0 - x_1*y_1*z_1);
a_2 = (C_000*x_1*z_1 - C_001*x_1*z_0 - C_010*x_1*z_1 + C_011*x_1*z_0 - C_100*x_0*z_1 + C_101*x_0*z_0 + C_110*x_0*z_1 - C_111*x_0*z_0)/(x_0*y_0*z_0 - x_0*y_0*z_1 - x_0*y_1*z_0 + x_0*y_1*z_1 - x_1*y_0*z_0 + x_1*y_0*z_1 + x_1*y_1*z_0 - x_1*y_1*z_1);
a_3 = (C_000*x_1*y_1 - C_001*x_1*y_1 - C_010*x_1*y_0 + C_011*x_1*y_0 - C_100*x_0*y_1 + C_101*x_0*y_1 + C_110*x_0*y_0 - C_111*x_0*y_0)/(x_0*y_0*z_0 - x_0*y_0*z_1 - x_0*y_1*z_0 + x_0*y_1*z_1 - x_1*y_0*z_0 + x_1*y_0*z_1 + x_1*y_1*z_0 - x_1*y_1*z_1);
a_4 = (-C_000*z_1 + C_001*z_0 + C_010*z_1 - C_011*z_0 + C_100*z_1 - C_101*z_0 - C_110*z_1 + C_111*z_0)/(x_0*y_0*z_0 - x_0*y_0*z_1 - x_0*y_1*z_0 + x_0*y_1*z_1 - x_1*y_0*z_0 + x_1*y_0*z_1 + x_1*y_1*z_0 - x_1*y_1*z_1);
a_5 = (-C_000*y_1 + C_001*y_1 + C_010*y_0 - C_011*y_0 + C_100*y_1 - C_101*y_1 - C_110*y_0 + C_111*y_0)/(x_0*y_0*z_0 - x_0*y_0*z_1 - x_0*y_1*z_0 + x_0*y_1*z_1 - x_1*y_0*z_0 + x_1*y_0*z_1 + x_1*y_1*z_0 - x_1*y_1*z_1);
a_6 = (-C_000*x_1 + C_001*x_1 + C_010*x_1 - C_011*x_1 + C_100*x_0 - C_101*x_0 - C_110*x_0 + C_111*x_0)/(x_0*y_0*z_0 - x_0*y_0*z_1 - x_0*y_1*z_0 + x_0*y_1*z_1 - x_1*y_0*z_0 + x_1*y_0*z_1 + x_1*y_1*z_0 - x_1*y_1*z_1);
a_7 = (C_000 - C_001 - C_010 + C_011 - C_100 + C_101 + C_110 - C_111)/(x_0*y_0*z_0 - x_0*y_0*z_1 - x_0*y_1*z_0 + x_0*y_1*z_1 - x_1*y_0*z_0 + x_1*y_0*z_1 + x_1*y_1*z_0 - x_1*y_1*z_1);
    
id_interp = (a_0 + a_1*x + a_2*y + a_3*z + a_4*x*y + a_5*x*z + a_6*y*z + a_7*x*y*z);

== matlab function ee_import_fem_maxwell/PMSM model1/invLUT /MATLAB Function3 ==
  data: x input; iq_interp output; y input; z input; data parameter
function iq_interp = fcn(x,y,z,data)

% iD = data.i_d;
iQ = data.i_q;
fD = data.phi_d;
fQ = data.phi_d;
TH = data.theta;

% Buscamos los vértices del cubo
if x<fD(1)
    index_x0 = 1;
    index_x1 = 1;
elseif x>fD(end)
    index_x0 = length(fD);
    index_x1 = length(fD);
else
    x_aux = find(fD <= x);
    index_x0 = x_aux(end);
    index_x1 = x_aux(end)+1;
end
x_0 = fD(index_x0);
x_1 = fD(index_x1);

if y<fQ(1)
    index_y0 = 1;
    index_y1 = 1;
elseif y>fQ(end)
    index_y0 = length(fQ);
    index_y1 = length(fQ);
else
    y_aux = find(fQ <= y);
    index_y0 = y_aux(end);
    index_y1 = y_aux(end)+1;
end
y_0 = fQ(index_y0);
y_1 = fQ(index_y1);

if z<TH(1)
    index_z0 = 1;
    index_z1 = 1;
elseif z>TH(end)
    index_z0 = length(TH);
    index_z1 = length(TH);
else
    z_aux = find(TH <= z);
    index_z0 = z_aux(end);
    index_z1 = z_aux(end)+1;
end
z_0 = TH(index_z0);
z_1 = TH(index_z1);

C_000 = iQ(index_x0, index_y0, index_z0);
C_001 = iQ(index_x0, index_y0, index_z1);
C_010 = iQ(index_x0, index_y1, index_z0);
C_011 = iQ(index_x0, index_y1, index_z1);
C_100 = iQ(index_x1, index_y0, index_z0);
C_101 = iQ(index_x1, index_y0, index_z1);
C_110 = iQ(index_x1, index_y1, index_z0);
C_111 = iQ(index_x1, index_y1, index_z1);

a_0 = (-C_000*x_1*y_1*z_1 + C_001*x_1*y_1*z_0 + C_010*x_1*y_0*z_1 - C_011*x_1*y_0*z_0 + C_100*x_0*y_1*z_1 - C_101*x_0*y_1*z_0 - C_110*x_0*y_0*z_1 + C_111*x_0*y_0*z_0)/(x_0*y_0*z_0 - x_0*y_0*z_1 - x_0*y_1*z_0 + x_0*y_1*z_1 - x_1*y_0*z_0 + x_1*y_0*z_1 + x_1*y_1*z_0 - x_1*y_1*z_1);
a_1 = (C_000*y_1*z_1 - C_001*y_1*z_0 - C_010*y_0*z_1 + C_011*y_0*z_0 - C_100*y_1*z_1 + C_101*y_1*z_0 + C_110*y_0*z_1 - C_111*y_0*z_0)/(x_0*y_0*z_0 - x_0*y_0*z_1 - x_0*y_1*z_0 + x_0*y_1*z_1 - x_1*y_0*z_0 + x_1*y_0*z_1 + x_1*y_1*z_0 - x_1*y_1*z_1);
a_2 = (C_000*x_1*z_1 - C_001*x_1*z_0 - C_010*x_1*z_1 + C_011*x_1*z_0 - C_100*x_0*z_1 + C_101*x_0*z_0 + C_110*x_0*z_1 - C_111*x_0*z_0)/(x_0*y_0*z_0 - x_0*y_0*z_1 - x_0*y_1*z_0 + x_0*y_1*z_1 - x_1*y_0*z_0 + x_1*y_0*z_1 + x_1*y_1*z_0 - x_1*y_1*z_1);
a_3 = (C_000*x_1*y_1 - C_001*x_1*y_1 - C_010*x_1*y_0 + C_011*x_1*y_0 - C_100*x_0*y_1 + C_101*x_0*y_1 + C_110*x_0*y_0 - C_111*x_0*y_0)/(x_0*y_0*z_0 - x_0*y_0*z_1 - x_0*y_1*z_0 + x_0*y_1*z_1 - x_1*y_0*z_0 + x_1*y_0*z_1 + x_1*y_1*z_0 - x_1*y_1*z_1);
a_4 = (-C_000*z_1 + C_001*z_0 + C_010*z_1 - C_011*z_0 + C_100*z_1 - C_101*z_0 - C_110*z_1 + C_111*z_0)/(x_0*y_0*z_0 - x_0*y_0*z_1 - x_0*y_1*z_0 + x_0*y_1*z_1 - x_1*y_0*z_0 + x_1*y_0*z_1 + x_1*y_1*z_0 - x_1*y_1*z_1);
a_5 = (-C_000*y_1 + C_001*y_1 + C_010*y_0 - C_011*y_0 + C_100*y_1 - C_101*y_1 - C_110*y_0 + C_111*y_0)/(x_0*y_0*z_0 - x_0*y_0*z_1 - x_0*y_1*z_0 + x_0*y_1*z_1 - x_1*y_0*z_0 + x_1*y_0*z_1 + x_1*y_1*z_0 - x_1*y_1*z_1);
a_6 = (-C_000*x_1 + C_001*x_1 + C_010*x_1 - C_011*x_1 + C_100*x_0 - C_101*x_0 - C_110*x_0 + C_111*x_0)/(x_0*y_0*z_0 - x_0*y_0*z_1 - x_0*y_1*z_0 + x_0*y_1*z_1 - x_1*y_0*z_0 + x_1*y_0*z_1 + x_1*y_1*z_0 - x_1*y_1*z_1);
a_7 = (C_000 - C_001 - C_010 + C_011 - C_100 + C_101 + C_110 - C_111)/(x_0*y_0*z_0 - x_0*y_0*z_1 - x_0*y_1*z_0 + x_0*y_1*z_1 - x_1*y_0*z_0 + x_1*y_0*z_1 + x_1*y_1*z_0 - x_1*y_1*z_1);
    
iq_interp = (a_0 + a_1*x + a_2*y + a_3*z + a_4*x*y + a_5*x*z + a_6*y*z + a_7*x*y*z);
